simulink model "motorServoSystem"  (R2016a)
settings: Solver=VariableStepAuto  StartTime=0.0  StopTime=5  RelTol=1e-3
values from neighbouring files (symbols this model uses):
  b = 3.7*10^-6    (= 3.7e-06)    [sysParameter.m]
  J = 8.5*10^(-6)    (= 8.5e-06)    [sysParameter.m]
  Kamp = 1    [sysParameter.m]
  Kff = 1    [sysParameter.m]
  Kpd = 0.09    [sysParameter.m]
  Kpi = 0    [sysParameter.m]
  Kpp = 2    [sysParameter.m]
  Kt = 4.24*10^-2    (= 0.0424)    [sysParameter.m]
  Kvd = 0.2    [sysParameter.m]
  Kvi = 0    [sysParameter.m]
  Kvp = 25    [sysParameter.m]
  Np = 150    [sysParameter.m]
  Nv = 100    [sysParameter.m]
  tau = 6.6    [sysParameter.m]
libraries: simulink x3
settings Model: Creator=yeeyoung  LastModifiedBy=yeeyoung
settings DataIOCC: SaveState=on

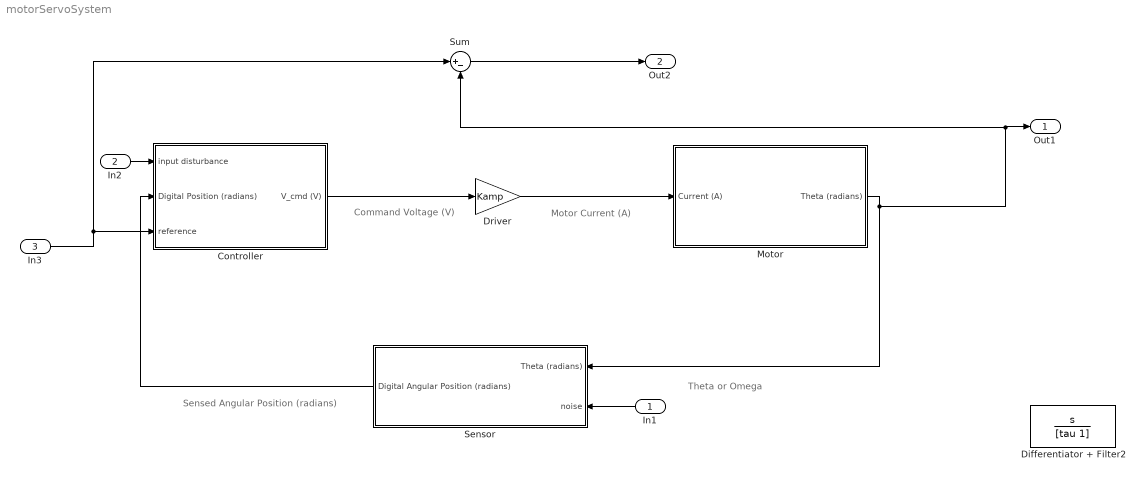
== system motorServoSystem ==
  note: Theta or Omega
  note: Sensed Angular Position (radians)
  note: Motor Current (A)
  note: Command Voltage (V)
  In1 : Inport
  In2 : Inport  Port=2
  In3 : Inport  Port=3
  Controller : Subsystem  TreatAsAtomicUnit=on
      settings: RTWFcnNameOpts=Use subsystem name  RTWFileNameOpts=Use function name
  Differentiator + Filter2 : TransferFcn  Numerator=[1 0]  Denominator=[tau 1]
  Driver : Gain  Gain=Kamp
  Motor : Subsystem  TreatAsAtomicUnit=on
      settings: RTWFcnNameOpts=Use subsystem name  RTWFileNameOpts=Use function name
  Sensor : Subsystem  TreatAsAtomicUnit=on
      settings: RTWFcnNameOpts=Use subsystem name  RTWFileNameOpts=Use function name
  Sum : Sum  Inputs=|+-
  Out1 : Outport
  Out2 : Outport  Port=2
  wires:
  Driver/1 -> Motor/1(Current (A))
  Sensor/1(Digital Angular Position (radians)) -> Controller/2(Digital Position (radians))
  In1/1 -> Sensor/2(noise)
  In2/1 -> Controller/1(input disturbance)
  In3/1 -> Sum/1, Controller/3(reference)
  Sum/1 -> Out2/1
  Motor/1(Theta (radians)) -> Sum/2, Out1/1, Sensor/1(Theta (radians))
  Controller/1(V_cmd (V)) -> Driver/1

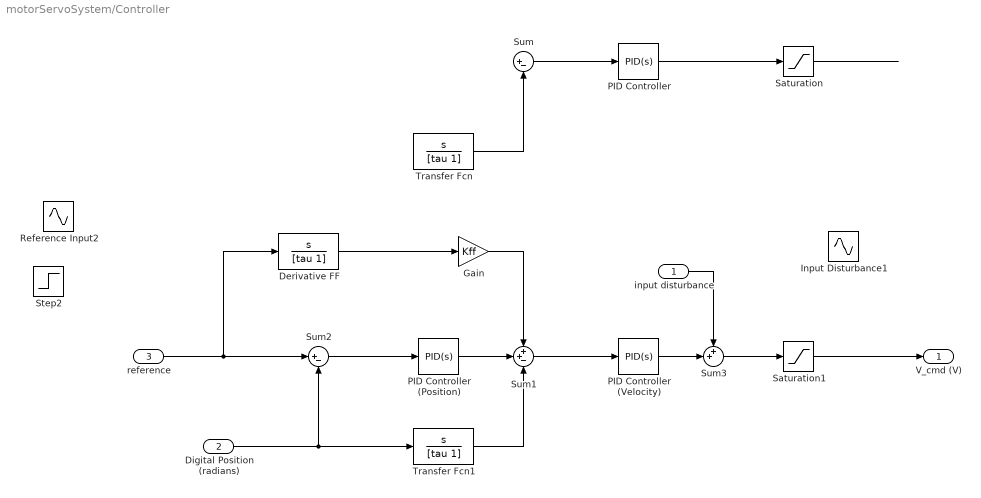
== system motorServoSystem/Controller ==
  input disturbance : Inport
  Digital Position (radians) : Inport  Port=2
  reference : Inport  Port=3
  Derivative FF : TransferFcn  Numerator=[1 0]  Denominator=[tau 1]
  Gain : Gain  Gain=Kff
  Input Disturbance1 : Sin  Amplitude=0  SampleTime=0
  PID Controller : simulink/Continuous/PID Controller  Controller=PID  TimeDomain=Continuous-time  SampleTime=-1  IntegratorMethod=Forward Euler  FilterMethod=Forward Euler  Form=Parallel  UseFilter=on  ControllerParametersSource=internal  P=Kvp  I=Kvi  D=Kvd  N=Nv  InitialConditionSource=internal  InitialConditionForIntegrator=0  InitialConditionForFilter=0  ExternalReset=none  LimitOutput=off  UpperSaturationLimit=inf  LowerSaturationLimit=-inf  LinearizeAsGain=on  AntiWindupMode=none  Kb=1  TrackingMode=off  Kt=1  PParamMin=[]  PParamMax=[]  IParamMin=[]  IParamMax=[]  DParamMin=[]  DParamMax=[]  NParamMin=[]  NParamMax=[]  KbParamMin=[]  KbParamMax=[]  KtParamMin=[]  KtParamMax=[]  POutMin=[]  POutMax=[]  IOutMin=[]  IOutMax=[]  DOutMin=[]  DOutMax=[]  NOutMin=[]  NOutMax=[]  KbOutMin=[]  KbOutMax=[]  KtOutMin=[]  KtOutMax=[]  IntegratorOutMin=[]  IntegratorOutMax=[]  FilterOutMin=[]  FilterOutMax=[]  SumOutMin=[]  SumOutMax=[]  SumI1OutMin=[]  SumI1OutMax=[]  SumI2OutMin=[]  SumI2OutMax=[]  SumI3OutMin=[]  SumI3OutMax=[]  SumDOutMin=[]  SumDOutMax=[]  SaturationOutMin=[]  SaturationOutMax=[]  IntegratorContinuousStateAttributes=''  IntegratorStateMustResolveToSignalObject=off  IntegratorRTWStateStorageClass=Auto  FilterContinuousStateAttributes=''  FilterStateMustResolveToSignalObject=off  FilterRTWStateStorageClass=Auto  DifferentiatorICPrevScaledInput=0  DifferentiatorOutMin=[]  DifferentiatorOutMax=[]
  PID Controller (Position) : simulink/Continuous/PID Controller  Controller=PID  TimeDomain=Continuous-time  SampleTime=-1  IntegratorMethod=Forward Euler  FilterMethod=Forward Euler  Form=Parallel  UseFilter=on  ControllerParametersSource=internal  P=Kpp  I=Kpi  D=Kpd  N=Np  InitialConditionSource=internal  InitialConditionForIntegrator=0  InitialConditionForFilter=0  ExternalReset=none  LimitOutput=off  UpperSaturationLimit=inf  LowerSaturationLimit=-inf  LinearizeAsGain=on  AntiWindupMode=none  Kb=1  TrackingMode=off  Kt=1  PParamMin=[]  PParamMax=[]  IParamMin=[]  IParamMax=[]  DParamMin=[]  DParamMax=[]  NParamMin=[]  NParamMax=[]  KbParamMin=[]  KbParamMax=[]  KtParamMin=[]  KtParamMax=[]  POutMin=[]  POutMax=[]  IOutMin=[]  IOutMax=[]  DOutMin=[]  DOutMax=[]  NOutMin=[]  NOutMax=[]  KbOutMin=[]  KbOutMax=[]  KtOutMin=[]  KtOutMax=[]  IntegratorOutMin=[]  IntegratorOutMax=[]  FilterOutMin=[]  FilterOutMax=[]  SumOutMin=[]  SumOutMax=[]  SumI1OutMin=[]  SumI1OutMax=[]  SumI2OutMin=[]  SumI2OutMax=[]  SumI3OutMin=[]  SumI3OutMax=[]  SumDOutMin=[]  SumDOutMax=[]  SaturationOutMin=[]  SaturationOutMax=[]  IntegratorContinuousStateAttributes=''  IntegratorStateMustResolveToSignalObject=off  IntegratorRTWStateStorageClass=Auto  FilterContinuousStateAttributes=''  FilterStateMustResolveToSignalObject=off  FilterRTWStateStorageClass=Auto  DifferentiatorICPrevScaledInput=0  DifferentiatorOutMin=[]  DifferentiatorOutMax=[]
  PID Controller (Velocity) : simulink/Continuous/PID Controller  Controller=PID  TimeDomain=Continuous-time  SampleTime=-1  IntegratorMethod=Forward Euler  FilterMethod=Forward Euler  Form=Parallel  UseFilter=on  ControllerParametersSource=internal  P=Kvp  I=Kvi  D=Kvd  N=Nv  InitialConditionSource=internal  InitialConditionForIntegrator=0  InitialConditionForFilter=0  ExternalReset=none  LimitOutput=off  UpperSaturationLimit=inf  LowerSaturationLimit=-inf  LinearizeAsGain=on  AntiWindupMode=none  Kb=1  TrackingMode=off  Kt=1  PParamMin=[]  PParamMax=[]  IParamMin=[]  IParamMax=[]  DParamMin=[]  DParamMax=[]  NParamMin=[]  NParamMax=[]  KbParamMin=[]  KbParamMax=[]  KtParamMin=[]  KtParamMax=[]  POutMin=[]  POutMax=[]  IOutMin=[]  IOutMax=[]  DOutMin=[]  DOutMax=[]  NOutMin=[]  NOutMax=[]  KbOutMin=[]  KbOutMax=[]  KtOutMin=[]  KtOutMax=[]  IntegratorOutMin=[]  IntegratorOutMax=[]  FilterOutMin=[]  FilterOutMax=[]  SumOutMin=[]  SumOutMax=[]  SumI1OutMin=[]  SumI1OutMax=[]  SumI2OutMin=[]  SumI2OutMax=[]  SumI3OutMin=[]  SumI3OutMax=[]  SumDOutMin=[]  SumDOutMax=[]  SaturationOutMin=[]  SaturationOutMax=[]  IntegratorContinuousStateAttributes=''  IntegratorStateMustResolveToSignalObject=off  IntegratorRTWStateStorageClass=Auto  FilterContinuousStateAttributes=''  FilterStateMustResolveToSignalObject=off  FilterRTWStateStorageClass=Auto  DifferentiatorICPrevScaledInput=0  DifferentiatorOutMin=[]  DifferentiatorOutMax=[]
  Reference Input2 : Sin  Amplitude=pi  Frequency=2*pi*5  SampleTime=0
  Saturation : Saturate  UpperLimit=6  LowerLimit=-6
  Saturation1 : Saturate  UpperLimit=6  LowerLimit=-6
  Step2 : Step  Time=0  After=pi  SampleTime=0
  Sum : Sum  Inputs=|+-
  Sum1 : Sum  Inputs=++-
  Sum2 : Sum  Inputs=|+-
  Sum3 : Sum  Inputs=++|
  Transfer Fcn : TransferFcn  Numerator=[1 0]  Denominator=[tau 1]
  Transfer Fcn1 : TransferFcn  Numerator=[1 0]  Denominator=[tau 1]
  V_cmd (V) : Outport
  wires:
  ? -> Sum/1
  Transfer Fcn/1 -> Sum/2
  Sum/1 -> PID Controller/1
  PID Controller/1 -> Saturation/1
  Sum1/1 -> PID Controller (Velocity)/1
  Sum2/1 -> PID Controller (Position)/1
  PID Controller (Velocity)/1 -> Sum3/2
  Sum3/1 -> Saturation1/1
  Derivative FF/1 -> Gain/1
  Gain/1 -> Sum1/1
  PID Controller (Position)/1 -> Sum1/2
  Transfer Fcn1/1 -> Sum1/3
  input disturbance/1 -> Sum3/1
  ? -> Transfer Fcn/1
  Saturation/1 -> ?
  reference/1 -> Sum2/1, Derivative FF/1
  Digital Position (radians)/1 -> Sum2/2, Transfer Fcn1/1
  Saturation1/1 -> V_cmd (V)/1

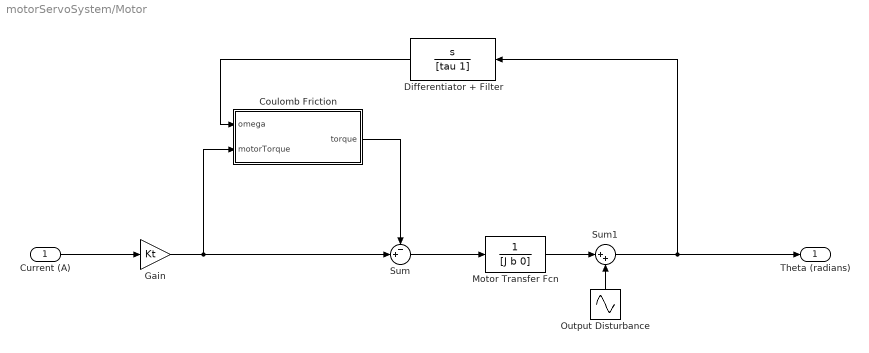
== system motorServoSystem/Motor ==
  Current (A) : Inport
  Coulomb Friction : MATLAB Function  TreatAsAtomicUnit=on
  Differentiator + Filter : TransferFcn  Numerator=[1 0]  Denominator=[tau 1]
  Gain : Gain  Gain=Kt
  Motor Transfer Fcn : TransferFcn  Denominator=[J b 0]
  Output Disturbance : Sin  Amplitude=0  SampleTime=0
  Sum : Sum  Inputs=-+|
  Sum1 : Sum  Inputs=|++
  Theta (radians) : Outport
  wires:
  Current (A)/1 -> Gain/1
  Gain/1 -> Coulomb Friction/2(motorTorque), Sum/2
  Sum/1 -> Motor Transfer Fcn/1
  Differentiator + Filter/1 -> Coulomb Friction/1(omega)
  Coulomb Friction/1(torque) -> Sum/1
  Output Disturbance/1 -> Sum1/2
  Motor Transfer Fcn/1 -> Sum1/1
  Sum1/1 -> Theta (radians)/1, Differentiator + Filter/1

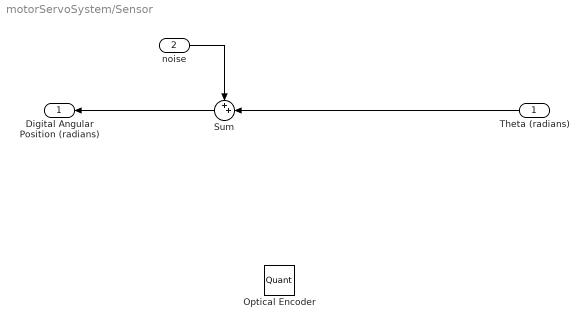
== system motorServoSystem/Sensor ==
  Theta (radians) : Inport
  noise : Inport  Port=2
  Optical Encoder : Quantizer  QuantizationInterval=2*pi/2000
  Sum : Sum  Inputs=++|
  Digital Angular Position (radians) : Outport
  wires:
  noise/1 -> Sum/1
  Sum/1 -> Digital Angular Position (radians)/1
  Theta (radians)/1 -> Sum/2

== matlab function motorServoSystem/Motor/Coulomb Friction ==
  data: omega input; torque output; motorTorque input
function torque = fcn(omega, motorTorque)
% coulombic friction cannont exceed the magnitude of motor torque and
% opposes attempted motion
% global CoulombicFrictionON Tf
CoulombicFrictionON = 1;

Tf = 5.6*10^-3;
% Fk = 0.05; % torque exerted by coulombic friction, kinetic friction
% Fs = 0.07; % torque exerted by static friction
if (CoulombicFrictionON == 0)
    torque = motorTorque - motorTorque;
else
%     if (abs(omega) < 1e-6) % if not moving, friction opposes attempted motion
%         if abs(motorTorque) < Fs
%             FF = abs(motorTorque); % and doesn't exceed the magnitude of the applied torque
%         else
%             FF = Fs;
%         end
%         torque = - FF * sign(motorTorque);
%         
%     else % if we are moving oppose the actual motion with kinetic friciton
%         torque = - Fk * sign(omega);
%     end
    if (abs(omega) >= 1e-6) % if motor is rotating
        torque = sign(omega) * Tf;
    else
        torque = omega/(1e-6)*Tf;
    end
end
end
